simulink model "Discrete_Model"  (R2021b)
settings: Solver=VariableStepAuto  StartTime=0.0  StopTime=10.0  RelTol=1e-3
values from neighbouring files (symbols this model uses):
  B_f = 10    [Discrete_Model_Parameters.m]
  B_r = 10    [Discrete_Model_Parameters.m]
  C_f = 1.9    [Discrete_Model_Parameters.m]
  C_m = 5    [Discrete_Model_Parameters.m]
  C_r = 1.9    [Discrete_Model_Parameters.m]
  C_r0 = 0.1    [Discrete_Model_Parameters.m]
  C_r2 = 0.2    [Discrete_Model_Parameters.m]
  D_f = 1    [Discrete_Model_Parameters.m]
  D_r = 1    [Discrete_Model_Parameters.m]
  delta_s = 0.1    [Discrete_Model_Parameters.m]
  FN_f = 54.5    [Discrete_Model_Parameters.m]
  FN_r = 43.6    [Discrete_Model_Parameters.m]
  I_z = 0.152    [Discrete_Model_Parameters.m]
  l_f = 2.5    [Discrete_Model_Parameters.m]
  l_r = 2    [Discrete_Model_Parameters.m]
  mass = 10    [Discrete_Model_Parameters.m]
  p_tv = 0    [Discrete_Model_Parameters.m]
settings Model: Creator=21738394  LastModifiedBy=21738394

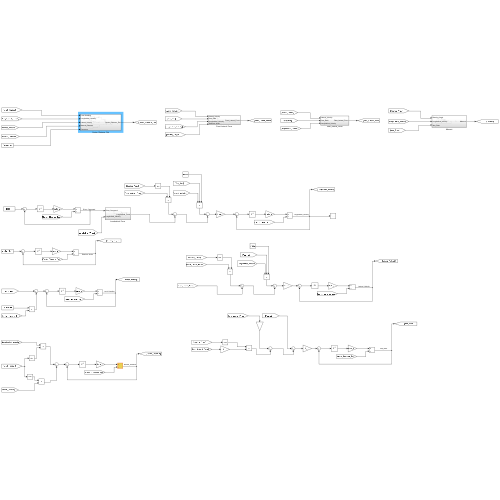
[thumbnail: Simulink's stored preview of the top-level diagram]
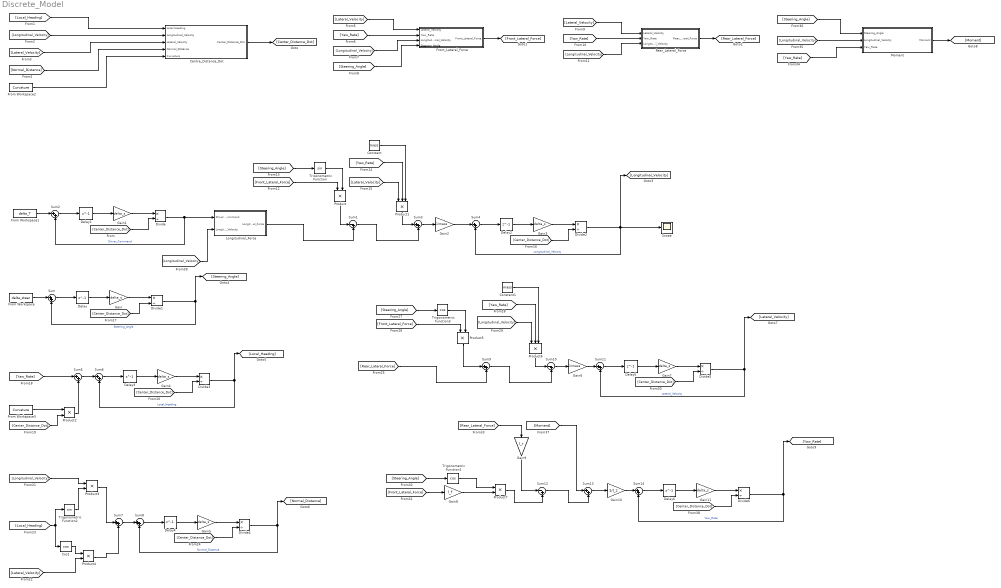
== system Discrete_Model ==
  Centre_Distance_Dot : Subsystem
  Constant : Constant  Value=mass
  Constant1 : Constant  Value=mass
  Cos1 : Trigonometry  Operator=cos
  Delay{,1..6} (7 alike) : Delay  DelayLength=1  InitialCondition=0
  Divide{,1..6} (7 alike) : Product  Inputs=*/
  From Workspace : FromWorkspace  VariableName=delta_steer
  From Workspace1 : FromWorkspace  VariableName=delta_T
  From Workspace2 : FromWorkspace  VariableName=Curvature
  From Workspace3 : FromWorkspace  VariableName=Curvature
  Front_Lateral_Force : Subsystem
  Gain{,1,3..5,7,11} (7 alike) : Gain  Gain=delta_s
  Gain10 : Gain  Gain=1/I_z
  Gain2 : Gain  Gain=1/mass
  Gain6 : Gain  Gain=1/mass
  Gain8 : Gain  Gain=l_f
  Gain9 : Gain  Gain=l_r
  Longitudinal_Force : Subsystem
  Moment : Subsystem
  Product{,2..5,7} (6 alike) : Product
  Product1 : Product  Inputs=3
  Product6 : Product  Inputs=3
  Rear_Lateral_Force : Subsystem
  Scope : Scope
  Sum{,2..9,11,13..14} (12 alike) : Sum  Inputs=|++
  Sum1 : Sum  Inputs=|-+
  Sum10 : Sum  Inputs=|-+
  Sum12 : Sum  Inputs=|-+
  Trigonometric Function : Trigonometry
  Trigonometric Function2 : Trigonometry
  Trigonometric Function3 : Trigonometry  Operator=cos
  Trigonometric Function4 : Trigonometry  Operator=cos
  wires:
  From Workspace/1 -> Sum/1
  Sum/1 -> Delay/1
  Delay/1 -> Gain/1
  From Workspace1/1 -> Sum2/1
  Delay1/1 -> Gain1/1
  Sum2/1 -> Delay1/1
  Gain1/1 -> Divide/1
  Centre_Distance_Dot/1(Center_Distance_Dot) -> [Center_Distance_Dot]
  [Center_Distance_Dot] -> Divide/2
  Divide/1 -> Sum2/2, Longitudinal_Force/1(Driver Command)  "Driver_Command"
  From Workspace2/1 -> Centre_Distance_Dot/5(Curvature)
  [Normal_Distance] -> Centre_Distance_Dot/4(Normal_Distance)
  [Lateral_Velocity] -> Centre_Distance_Dot/3(Lateral_Velocity)
  [Longitudinal_Velocity] -> Centre_Distance_Dot/2(Longitudinal_Velocity)
  [Local_Heading] -> Centre_Distance_Dot/1(Local Heading)
  [Lateral_Velocity] -> Front_Lateral_Force/1(Lateral_Velocity)
  [Yaw_Rate] -> Front_Lateral_Force/2(Yaw_Rate)
  [Longitudinal_Velocity] -> Front_Lateral_Force/3(Longitudinal_Velocity)
  [Steering_Angle] -> Front_Lateral_Force/4(Steering_Angle)
  Front_Lateral_Force/1(Front_Lateral_Force) -> [Front_Lateral_Force]
  [Longitudinal_Velocity] -> Rear_Lateral_Force/3(Longitudinal_Velocity)
  [Yaw_Rate] -> Rear_Lateral_Force/2("Yaw_Rate ")
  [Lateral_Velocity] -> Rear_Lateral_Force/1(Lateral_Velocity)
  Rear_Lateral_Force/1(Rear_Lateral_Force) -> [Rear_Lateral_Force]
  Longitudinal_Force/1(Longitudinal_Force) -> Sum1/2
  [Steering_Angle] -> Trigonometric Function/1
  Trigonometric Function/1 -> Product/2
  [Front_Lateral_Force] -> Product/1
  Product/1 -> Sum1/1
  Sum1/1 -> Sum3/2
  [Lateral_Velocity] -> Product1/1
  [Yaw_Rate] -> Product1/2
  Constant/1 -> Product1/3
  Product1/1 -> Sum3/1
  Sum3/1 -> Gain2/1
  Gain/1 -> Divide1/1
  [Center_Distance_Dot] -> Divide1/2
  Delay2/1 -> Gain3/1
  Sum4/1 -> Delay2/1
  Divide2/1 -> Scope/1, Sum4/2, [Longitudinal_Velocity]  "Longitudinal_Velocity"
  [Center_Distance_Dot] -> Divide2/2
  Gain3/1 -> Divide2/1
  Gain2/1 -> Sum4/1
  Divide1/1 -> [Steering_Angle], Sum/2  "Steering_Angle"
  [Yaw_Rate] -> Sum5/1
  [Center_Distance_Dot] -> Product2/2
  From Workspace3/1 -> Product2/1
  Product2/1 -> Sum5/2
  Delay3/1 -> Gain4/1
  Sum6/1 -> Delay3/1
  Divide3/1 -> Sum6/2, [Local_Heading]  "Local_Heading"
  [Center_Distance_Dot] -> Divide3/2
  Gain4/1 -> Divide3/1
  Sum5/1 -> Sum6/1
  [Local_Heading] -> Cos1/1, Trigonometric Function2/1
  [Lateral_Velocity] -> Product4/2
  Cos1/1 -> Product4/1
  Trigonometric Function2/1 -> Product3/2
  [Longitudinal_Velocity] -> Product3/1
  Product3/1 -> Sum7/1
  Product4/1 -> Sum7/2
  [Center_Distance_Dot] -> Divide4/2
  Divide4/1 -> Sum8/2, [Normal_Distance]  "Normal_Distance"
  Sum7/1 -> Sum8/1
  Gain5/1 -> Divide4/1
  Delay4/1 -> Gain5/1
  Sum8/1 -> Delay4/1
  [Steering_Angle] -> Trigonometric Function3/1
  [Yaw_Rate] -> Product6/2
  Constant1/1 -> Product6/3
  Sum9/1 -> Sum10/2
  [Rear_Lateral_Force] -> Sum9/2
  Sum10/1 -> Gain6/1
  [Longitudinal_Velocity] -> Product6/1
  Product6/1 -> Sum10/1
  Product5/1 -> Sum9/1
  Gain7/1 -> Divide5/1
  Gain6/1 -> Sum11/1
  [Front_Lateral_Force] -> Product5/1
  [Center_Distance_Dot] -> Divide5/2
  Divide5/1 -> Sum11/2, [Lateral_Velocity]  "Lateral_Velocity"
  Sum11/1 -> Delay5/1
  Delay5/1 -> Gain7/1
  Trigonometric Function3/1 -> Product5/2
  [Steering_Angle] -> Trigonometric Function4/1
  Trigonometric Function4/1 -> Product7/1
  [Front_Lateral_Force] -> Gain8/1
  Gain8/1 -> Product7/2
  Product7/1 -> Sum12/2
  [Rear_Lateral_Force] -> Gain9/1
  Gain9/1 -> Sum12/1
  Sum12/1 -> Sum13/2
  [Steering_Angle] -> Moment/1(Steering_Angle)
  [Longitudinal_Velocity] -> Moment/2(Longitudinal_Velocity)
  [Yaw_Rate] -> Moment/3(Yaw_Rate)
  Moment/1(Moment) -> [Moment]
  [Moment] -> Sum13/1
  Delay6/1 -> Gain11/1
  Gain10/1 -> Sum14/1
  Gain11/1 -> Divide6/1
  Sum14/1 -> Delay6/1
  [Center_Distance_Dot] -> Divide6/2
  Divide6/1 -> Sum14/2, [Yaw_Rate]  "Yaw_Rate"
  Sum13/1 -> Gain10/1
  [Longitudinal_Velocity] -> Longitudinal_Force/2(Longitudinal_Velocity)

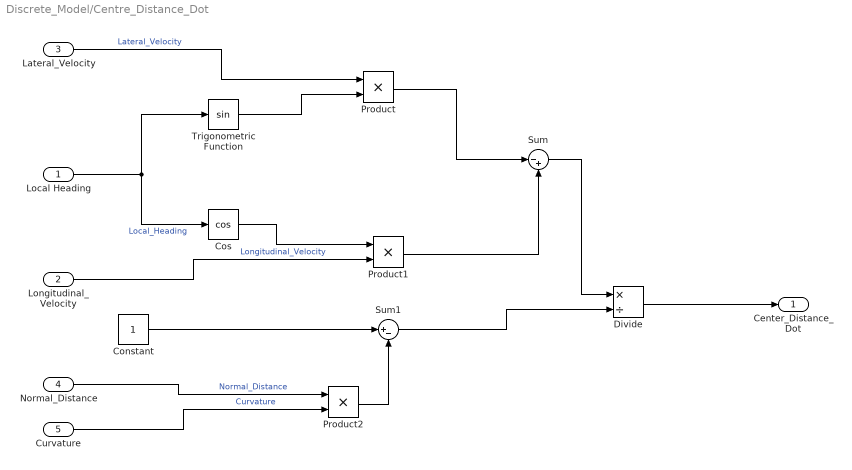
== system Discrete_Model/Centre_Distance_Dot ==
  Local Heading : Inport
  Longitudinal_Velocity : Inport  Port=2
  Lateral_Velocity : Inport  Port=3
  Normal_Distance : Inport  Port=4
  Curvature : Inport  Port=5
  Constant : Constant
  Cos : Trigonometry  Operator=cos
  Divide : Product  Inputs=*/
  Product : Product
  Product1 : Product
  Product2 : Product
  Sum : Sum  Inputs=|-+
  Sum1 : Sum  Inputs=|+-
  Trigonometric Function : Trigonometry
  Center_Distance_Dot : Outport
  wires:
  Local Heading/1 -> Trigonometric Function/1, Cos/1  "Local_Heading"
  Lateral_Velocity/1 -> Product/1  "Lateral_Velocity"
  Trigonometric Function/1 -> Product/2
  Longitudinal_Velocity/1 -> Product1/2  "Longitudinal_Velocity"
  Cos/1 -> Product1/1
  Product/1 -> Sum/1
  Product1/1 -> Sum/2
  Sum/1 -> Divide/1
  Constant/1 -> Sum1/1
  Normal_Distance/1 -> Product2/1  "Normal_Distance"
  Curvature/1 -> Product2/2  "Curvature"
  Product2/1 -> Sum1/2
  Sum1/1 -> Divide/2
  Divide/1 -> Center_Distance_Dot/1

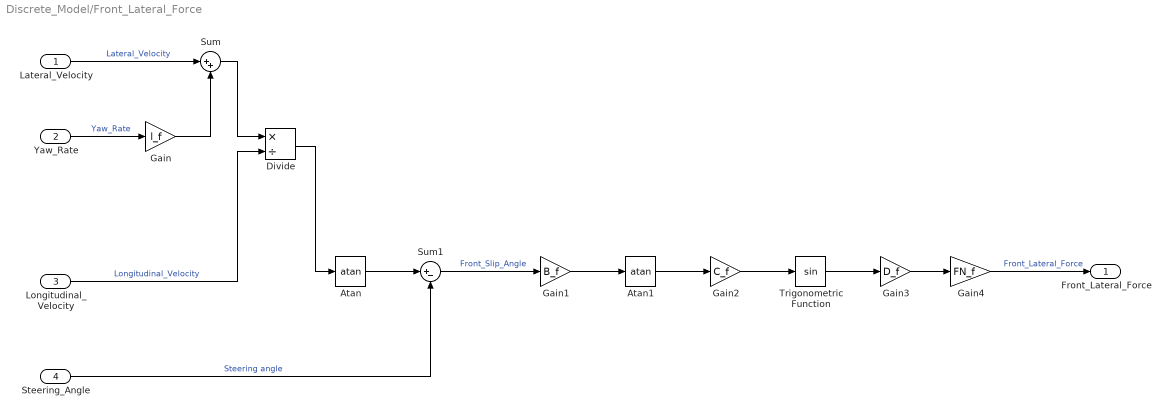
== system Discrete_Model/Front_Lateral_Force ==
  Lateral_Velocity : Inport
  Yaw_Rate : Inport  Port=2
  Longitudinal_Velocity : Inport  Port=3
  Steering_Angle : Inport  Port=4
  Atan : Trigonometry  Operator=atan
  Atan1 : Trigonometry  Operator=atan
  Divide : Product  Inputs=*/
  Gain : Gain  Gain=l_f
  Gain1 : Gain  Gain=B_f
  Gain2 : Gain  Gain=C_f
  Gain3 : Gain  Gain=D_f
  Gain4 : Gain  Gain=FN_f
  Sum : Sum  Inputs=|++
  Sum1 : Sum  Inputs=|+-
  Trigonometric Function : Trigonometry
  Front_Lateral_Force : Outport
  wires:
  Lateral_Velocity/1 -> Sum/1  "Lateral_Velocity"
  Yaw_Rate/1 -> Gain/1  "Yaw_Rate"
  Gain/1 -> Sum/2
  Sum/1 -> Divide/1
  Longitudinal_Velocity/1 -> Divide/2  "Longitudinal_Velocity"
  Steering_Angle/1 -> Sum1/2  "Steering angle"
  Divide/1 -> Atan/1
  Atan/1 -> Sum1/1
  Sum1/1 -> Gain1/1  "Front_Slip_Angle"
  Gain1/1 -> Atan1/1
  Atan1/1 -> Gain2/1
  Gain2/1 -> Trigonometric Function/1
  Trigonometric Function/1 -> Gain3/1
  Gain3/1 -> Gain4/1
  Gain4/1 -> Front_Lateral_Force/1  "Front_Lateral_Force"

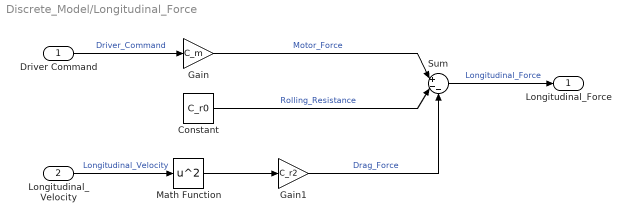
== system Discrete_Model/Longitudinal_Force ==
  Driver Command : Inport
  Longitudinal_Velocity : Inport  Port=2
  Constant : Constant  Value=C_r0
  Gain : Gain  Gain=C_m
  Gain1 : Gain  Gain=C_r2
  Math Function : Math  Operator=square  SaturateOnIntegerOverflow=on
  Sum : Sum  Inputs=|+--
  Longitudinal_Force : Outport
  wires:
  Driver Command/1 -> Gain/1  "Driver_Command"
  Gain/1 -> Sum/1  "Motor_Force"
  Constant/1 -> Sum/2  "Rolling_Resistance"
  Gain1/1 -> Sum/3  "Drag_Force"
  Longitudinal_Velocity/1 -> Math Function/1  "Longitudinal_Velocity"
  Math Function/1 -> Gain1/1
  Sum/1 -> Longitudinal_Force/1  "Longitudinal_Force"

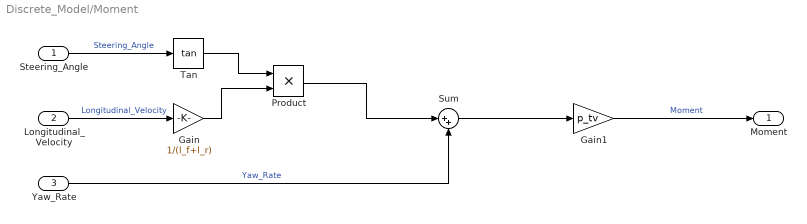
== system Discrete_Model/Moment ==
  Steering_Angle : Inport
  Longitudinal_Velocity : Inport  Port=2
  Yaw_Rate : Inport  Port=3
  Gain : Gain  Gain=1/(l_f+l_r)
  Gain1 : Gain  Gain=p_tv
  Product : Product
  Sum : Sum  Inputs=|++
  Tan : Trigonometry  Operator=tan
  Moment : Outport
  wires:
  Steering_Angle/1 -> Tan/1  "Steering_Angle"
  Tan/1 -> Product/1
  Gain/1 -> Product/2
  Longitudinal_Velocity/1 -> Gain/1  "Longitudinal_Velocity"
  Product/1 -> Sum/1
  Yaw_Rate/1 -> Sum/2  "Yaw_Rate"
  Sum/1 -> Gain1/1
  Gain1/1 -> Moment/1  "Moment"

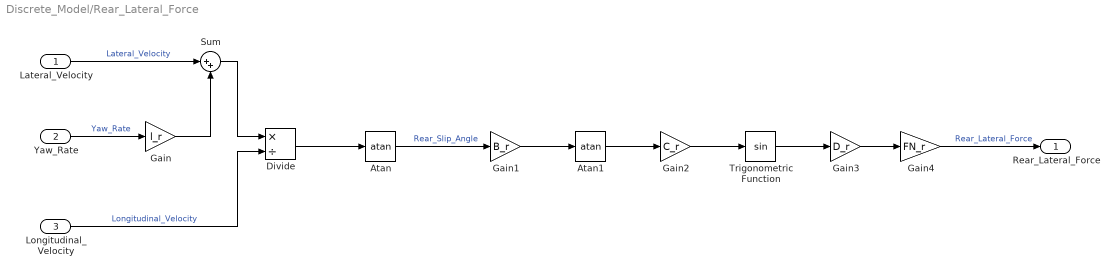
== system Discrete_Model/Rear_Lateral_Force ==
  Lateral_Velocity : Inport
  "Yaw_Rate " : Inport  Port=2
  Longitudinal_Velocity : Inport  Port=3
  Atan : Trigonometry  Operator=atan
  Atan1 : Trigonometry  Operator=atan
  Divide : Product  Inputs=*/
  Gain : Gain  Gain=l_r
  Gain1 : Gain  Gain=B_r
  Gain2 : Gain  Gain=C_r
  Gain3 : Gain  Gain=D_r
  Gain4 : Gain  Gain=FN_r
  Sum : Sum  Inputs=|++
  Trigonometric Function : Trigonometry
  Rear_Lateral_Force : Outport
  wires:
  Lateral_Velocity/1 -> Sum/1  "Lateral_Velocity"
  "Yaw_Rate "/1 -> Gain/1  "Yaw_Rate"
  Gain/1 -> Sum/2
  Sum/1 -> Divide/1
  Longitudinal_Velocity/1 -> Divide/2  "Longitudinal_Velocity"
  Divide/1 -> Atan/1
  Atan/1 -> Gain1/1  "Rear_Slip_Angle"
  Gain1/1 -> Atan1/1
  Atan1/1 -> Gain2/1
  Gain2/1 -> Trigonometric Function/1
  Trigonometric Function/1 -> Gain3/1
  Gain3/1 -> Gain4/1
  Gain4/1 -> Rear_Lateral_Force/1  "Rear_Lateral_Force"
